simulink model "hopfiled_model"  (R2022b)
settings: Solver=VariableStepAuto  StartTime=0.0  StopTime=10  RelTol=1e-3
settings Model: Creator=Lenovo  LastModifiedBy=Lenovo

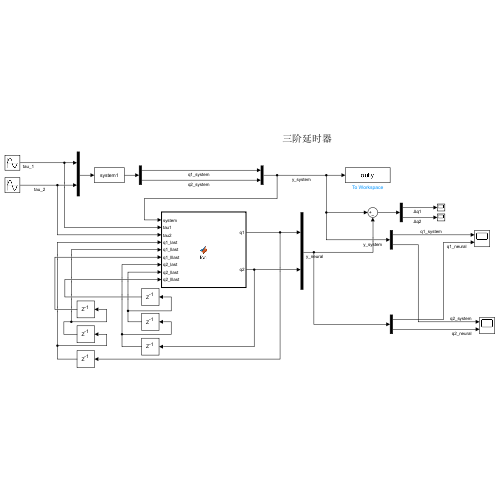
[thumbnail: Simulink's stored preview of the top-level diagram]
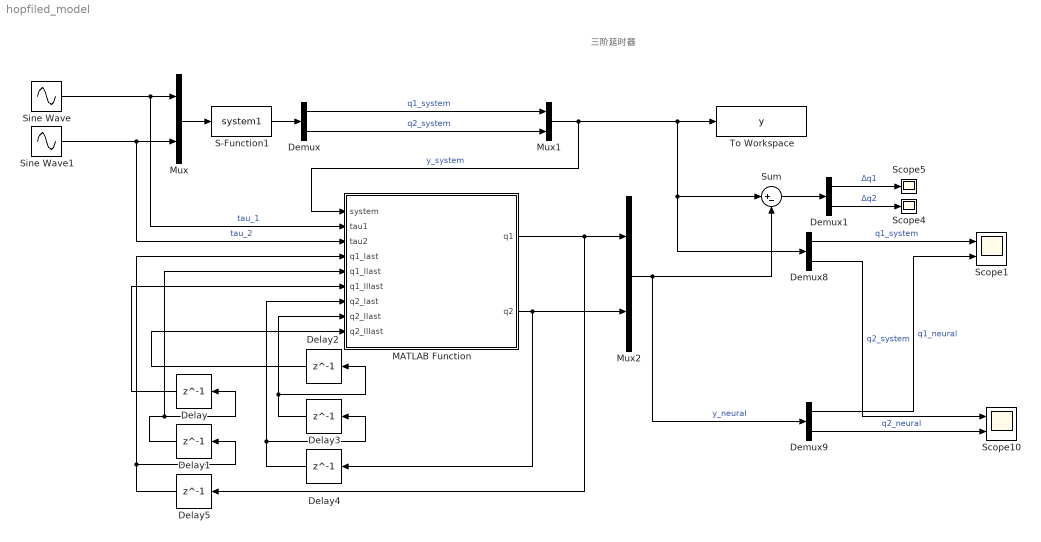
== system hopfiled_model ==
  note: 三阶延时器
  Delay{,1..5} (6 alike) : Delay  DelayLength=1  InitialCondition=0  SampleTime=0.001
  Demux{,1,8..9} (4 alike) : Demux  Outputs=2
  MATLAB Function : MATLAB Function  TreatAsAtomicUnit=on
  Mux : Mux  Inputs=2
  Mux1 : Mux  Inputs=2
  Mux2 : Mux  Inputs=2
  S-Function1 : S-Function  FunctionName=system1  SFunctionDeploymentMode=off  EnableBusSupport=off
  Scope1 : Scope  NumInputPorts=2
  Scope10 : Scope  NumInputPorts=2
  Scope4 : Scope
  Scope5 : Scope
  Sine Wave : Sin  SampleTime=0
  Sine Wave1 : Sin  SampleTime=0
  Sum : Sum  Inputs=|+-
  To Workspace : ToWorkspace  VariableName=y  SaveFormat=Timeseries  SampleTime=0.001
  wires:
  Mux/1 -> S-Function1/1
  Demux1/1 -> Scope5/1  "Δq1"
  Demux/1 -> Mux1/1  "q1_system"
  Sine Wave/1 -> MATLAB Function/2(tau1), Mux/1  "tau_1"
  Demux9/1 -> Scope1/2  "q1_neural"
  S-Function1/1 -> Demux/1
  Demux9/2 -> Scope10/2  "q2_neural"
  Demux/2 -> Mux1/2  "q2_system"
  Demux8/1 -> Scope1/1  "q1_system"
  Mux1/1 -> MATLAB Function/1(system), Demux8/1, Sum/1, To Workspace/1  "y_system"
  Sine Wave1/1 -> MATLAB Function/3(tau2), Mux/2  "tau_2"
  Demux8/2 -> Scope10/1  "q2_system"
  Demux1/2 -> Scope4/1  "Δq2"
  Sum/1 -> Demux1/1
  MATLAB Function/1(q1) -> Delay5/1, Mux2/1
  MATLAB Function/2(q2) -> Delay4/1, Mux2/2
  Delay4/1 -> Delay3/1, MATLAB Function/7(q2_last)
  Delay3/1 -> Delay2/1, MATLAB Function/8(q2_llast)
  Delay2/1 -> MATLAB Function/9(q2_lllast)
  Delay5/1 -> Delay1/1, MATLAB Function/4(q1_last)
  Delay1/1 -> Delay/1, MATLAB Function/5(q1_llast)
  Delay/1 -> MATLAB Function/6(q1_lllast)
  Mux2/1 -> Sum/2, Demux9/1  "y_neural"

== matlab function hopfiled_model/MATLAB Function ==
  settings: updateMethod=DISCRETE  sampleTime=0.01
  data: system input; tau1 input; q1 output; tau2 input; q1_last input; q1_llast input; q1_lllast input; q2_last input; q2_llast input; q2_lllast input; q2 output
function [q1, q2] = fcn(system, tau1, tau2, q1_last, q1_llast, q1_lllast, q2_last, q2_llast, q2_lllast)
    % fcn - 基于Hopfield神经网络的训练与预测函数，使用梯度下降法更新权重，并设置更新次数
    % 输入：
    %   system     - 目标系统的输出（2x1向量）
    %   tau1, tau2 - 外部输入信号（力矩）
    %   q1_last, q2_last - 上一时刻的输出
    %   q1_llast, q2_llast - 上上时刻的输出
    %   q1_lllast, q2_lllast - 上三时刻的输出
    % 输出：
    %   q1, q2 - 神经网络的预测输出

    % 初始化输入向量，包含历史输出和外部输入
    input = [q1_lllast; q2_lllast; q1_llast; q2_llast; q1_last; q2_last; tau1; tau2];
    
    % 初始化参数
    persistent count W eta eta_initial decay_rate decay_steps max_iter
    if isempty(count)
        count = 0;  % 计数器，用于控制更新
    end
    if isempty(W)
        W = zeros(8, 2);  % 8个输入对应2个输出（q1, q2）
    end
    if isempty(eta_initial)
        eta_initial = 0.0000014;  % 初始学习率
    end
    if isempty(decay_rate)
        decay_rate = 0.9;  % 衰减率
    end
    if isempty(decay_steps)
        decay_steps = 50;  % 每50步衰减一次学习率
    end
    if isempty(max_iter)
        max_iter = 10000;  % 最大迭代次数（梯度下降更新次数）
    end

    % 更新学习率（使用指数衰减方式）
    count = count + 1;
    eta = eta_initial * (decay_rate ^ (count / decay_steps));  % 计算衰减后的学习率

    % 计算目标输出与预测输出之间的误差
    error_last = system - W' * input;  % 初始误差计算

    % 执行梯度下降
    for i = 1:max_iter
        % 计算梯度：损失函数关于权重的梯度（均方误差）
        grad = -input * error_last';  % 梯度：对每个权重的贡献
        
        % 更新权重：梯度下降法
        W = W - eta * grad;

        % 每次迭代后计算L2范数并进行归一化
        W_norm = norm(W, 'fro');  % Frobenius范数：所有元素的平方和的平方根
        if W_norm > 1e-6  % 避免极小的数值误差
            W = W / W_norm;  % 归一化
        end
        
        % 计算当前误差
        error_curr = system - W' * input;
        
        % 如果误差收敛（误差的L2范数小于阈值），提前终止
        if norm(error_curr) < 1e-6
            break;  % 提前终止训练
        end

        % 如果误差变化非常小，则提前停止迭代（改进的提前终止条件）
        if norm(error_curr - error_last) < 1e-6
            break;
        end

        % 更新误差
        error_last = error_curr;
    end

    % 使用Hopfield网络的更新规则进行预测
    q = W' * input;  % 预测输出

    % 输出神经网络的预测结果
    q1 = q(1);  % 第一个输出对应q1
    q2 = q(2);  % 第二个输出对应q2
end
